simulink model "With_Noise_Assignment4"  (R2021a)
settings: Solver=VariableStepAuto  StartTime=0.0  StopTime=20.0  RelTol=1e-3
values from neighbouring files (symbols this model uses):
  A = [0 0 1 0 ... (first row only)    [Support_Script.m]    (also in Support_Script_with_noise.m)
  B = [0; 0; 1/mc; 1/(L*mc)]    [Support_Script.m]    (also in Support_Script_with_noise.m)
  C = [1 0 0 0]    [Support_Script.m]    (also in Support_Script_with_noise.m)
  Kr = lqr(A,B,Q1,R1)    [Support_Script.m]    (also in Support_Script_with_noise.m)
undefined symbols (not defined in the file or in its folder): Kf
libraries: simulink x1
settings Model: Creator=jai_bhawani  LastModifiedBy=jai_bhawani

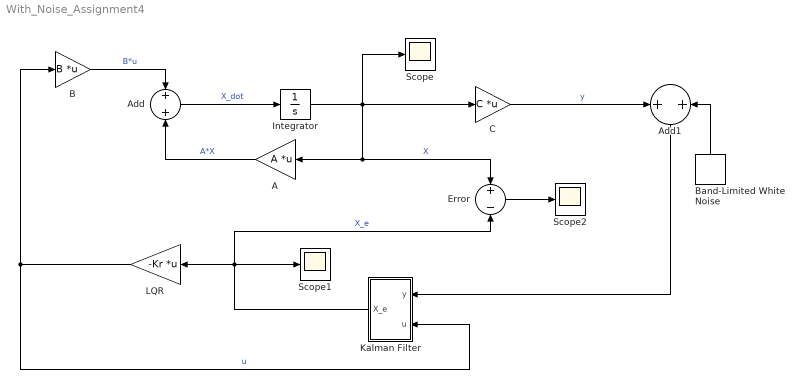
== system With_Noise_Assignment4 ==
  A : Gain  Gain=A  Multiplication=Matrix(K*u)
  Add : Sum
  Add1 : Sum
  B : Gain  Gain=B  Multiplication=Matrix(K*u)
  Band-Limited White Noise : simulink/Sources/Band-Limited White Noise  Cov=0.00005  Ts=0.1  seed=[9]
  C : Gain  Gain=C  Multiplication=Matrix(K*u)
  Error : Sum  Inputs=+-
  Integrator : Integrator  InitialCondition=[0; (10*pi)/180; 0; 0]  WrappedStateUpperValue=[inf;2*pi;inf;inf]  WrappedStateLowerValue=[-inf;0;-inf;-inf]
  Kalman Filter : Subsystem
  LQR : Gain  Gain=-Kr  Multiplication=Matrix(K*u)
  Scope : Scope
  Scope1 : Scope
  Scope2 : Scope
  wires:
  Error/1 -> Scope2/1
  A/1 -> Add/2  "A*X"
  Kalman Filter/1(X_e) -> Scope1/1, Error/2, LQR/1  "X_e"
  Add/1 -> Integrator/1  "X_dot"
  LQR/1 -> Kalman Filter/2(u), B/1  "u"
  C/1 -> Add1/1  "y"
  Band-Limited White Noise/1 -> Add1/2
  Integrator/1 -> C/1, Error/1, A/1, Scope/1  "X"
  B/1 -> Add/1  "B*u"
  Add1/1 -> Kalman Filter/1(y)

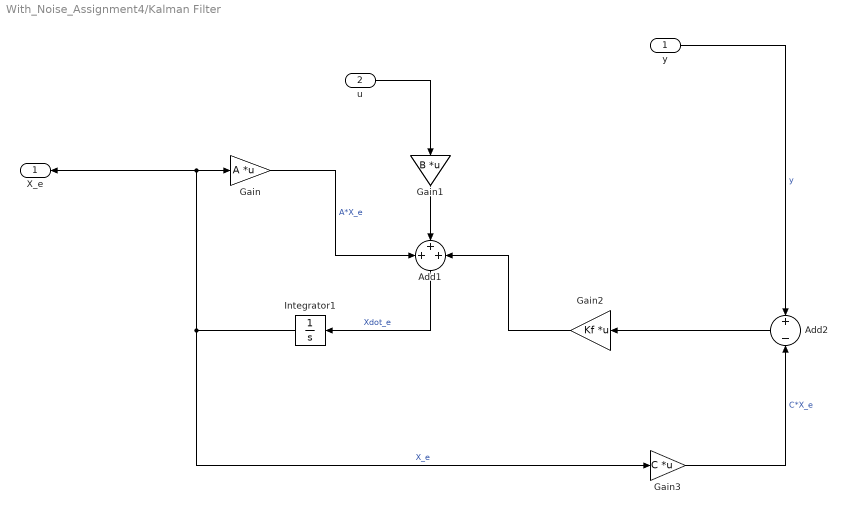
== system With_Noise_Assignment4/Kalman Filter ==
  y : Inport
  u : Inport  Port=2
  Add1 : Sum  Inputs=+++
  Add2 : Sum  Inputs=+-
  Gain : Gain  Gain=A  Multiplication=Matrix(K*u)
  Gain1 : Gain  Gain=B  Multiplication=Matrix(K*u)
  Gain2 : Gain  Gain=Kf  Multiplication=Matrix(K*u)
  Gain3 : Gain  Gain=C  Multiplication=Matrix(K*u)
  Integrator1 : Integrator  InitialCondition=[0;(10*pi)/180;0;0]
  X_e : Outport
  wires:
  Add1/1 -> Integrator1/1  "Xdot_e"
  Integrator1/1 -> Gain3/1, Gain/1, X_e/1  "X_e"
  u/1 -> Gain1/1
  Add2/1 -> Gain2/1
  y/1 -> Add2/1  "y"
  Gain3/1 -> Add2/2  "C*X_e"
  Gain1/1 -> Add1/2
  Gain2/1 -> Add1/3
  Gain/1 -> Add1/1  "A*X_e"
